simulink model "ScenarioAnalysis"  (R2022a)
settings: Solver=FixedStepDiscrete  StartTime=0.0  StopTime=10.0  RelTol=1e-3
model workspace (MAT data in the model file):
  firstWarning = 1
  originalScenarioChecksum = '40B3C482BC2D2C68EC305C2064A27088'
libraries: drivingscenarioandsensors x2
settings Model: Creator=Jim T  LastModifiedBy=11064

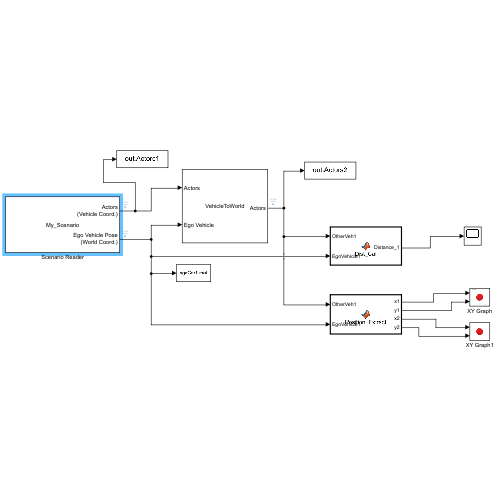
[thumbnail: Simulink's stored preview of the top-level diagram]
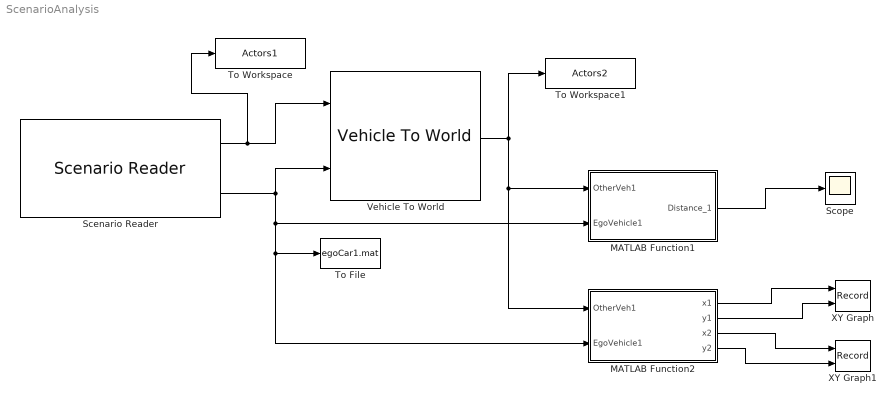
== system ScenarioAnalysis ==
  MATLAB Function1 : MATLAB Function  TreatAsAtomicUnit=on
  MATLAB Function2 : MATLAB Function  TreatAsAtomicUnit=on
  Scenario Reader : drivingscenarioandsensors/Scenario Reader  ScenarioSource=From file  ScenarioFileName=My_Scenario.mat  ScenarioVariableName=scenario  OutputCoordinateSystem=Vehicle coordinates  EgoVehicleSource=Scenario  EgoVehicleActorID=1  OrientVehiclesOnRoad=off  OutputEgoVehiclePose=on  OutputEgoVehicleState=off  SampleTime=0.1  LaneBoundaryOutput=None  LaneBoundaryDistance=0:0.5:9.5  LaneBoundaryLocation=Center of lane markings  BusNameSource=Auto  BusName=BusActors  BusNumActorsSource=Scenario  BusNumActors=100  BusName2Source=Auto  BusName2=BusLaneBoundaries  BusNumLaneBoundariesSource=Scenario  BusNumLaneBoundaries=10  BusName3Source=Auto  BusName3=BusEgoActor  BusName4Source=Auto  BusName4=BusEgoState  ShowCoordinateLabels=on  SimulateUsing=Interpreted execution
  Scope : Scope
  To File : ToFile  Filename=egoCar1.mat  SaveFormat=Timeseries
  To Workspace : ToWorkspace  VariableName=Actors1  SaveFormat=Timeseries  SampleTime=-1
  To Workspace1 : ToWorkspace  VariableName=Actors2  SaveFormat=Timeseries  SampleTime=-1
  Vehicle To World : drivingscenarioandsensors/Vehicle To World  BusNameSource=Auto  BusName=BusVehicleToWorldActors  SimulateUsing=Interpreted execution
      settings: SourceProductBaseCode=DR
  XY Graph : Record  FileSettingsInternal="{\"entries\":[{\"content\":{\"excelSettings\":{\"content\":{},\"type\":\"Streamout.ExcelSettings\"}},\"type\":\"Streamout.FileSettingStorage\",\"uuid\":\"b51cf517-17e0-4542-acce-b7d9d2cd1a5a\"}],\"packageUris\":[\"http://schema.mathworks.com/mf0/streamout_blocks/R2020a\"],\"version\":\"1.0\"}"  Layout=[1 1]  SignalsInternal="{\"entries\":[{\"content\":{\"signals\":[{\"content\":{\"blockPath\":[\"ScenarioAnalysis/XY Graph\"],\"channel\":[],\"dimensions\":[1],\"domain\":\"ScenarioAnalysis/XY Graph\",\"lineColor\":\"#a2142f\",\"plots\":[1],\"port\":1,\"sid\":[],\"signalID\":35,\"signalName\":\"MATLAB Function2:1\"},\"type\":\"RecordBlkView.Signal\",\"uuid\":\"04b8474e-6d3d-4901-9223-983ad539c10e\"},{\"content\":{\"blockPath\":[\"ScenarioAnalysis/XY Graph\"],\"channel\":[],\"dimensions\":[1],\"domain\":\"ScenarioAnalysis/XY Graph\",\"lineColor\":\"#139fff\",\"plots\":[1],\"port\":2,\"sid\":[],\"signalID\":38,\"signalName\":\"MATLAB Function2:2\"},\"type\":\"RecordBlkView.Signal\",\"uuid\":\"012edd8f-518d-447d-b22c-72d910c1f49f\"}]},\"type\":\"RecordBlkView.InputSignals\",\"uuid\":\"3fa3c5aa-3a4d-44aa-9af0-7d29b792f97e\"}],\"packageUris\":[\"http://schema.mathworks.com/mf0/streamout_blocks/R2020a\"],\"version\":\"1.0\"}"  VisualizationBindings="{\"xyplotplugin\":{\"info\":[{\"series\":[{\"bindingParametersList\":[{\"parameter\":\"X-Axis\",\"signalID\":35,\"signalName\":\"MATLAB Function2:1\"},{\"parameter\":\"Y-Axis\",\"signalID\":38,\"signalName\":\"MATLAB Function2:2\"}],\"seriesID\":38687}],\"subplotID\":1}]}}"  CompatibilityTag=XY
  XY Graph1 : Record  FileSettingsInternal="{\"entries\":[{\"content\":{\"excelSettings\":{\"content\":{},\"type\":\"Streamout.ExcelSettings\"}},\"type\":\"Streamout.FileSettingStorage\",\"uuid\":\"6fa187cc-d8dd-4e57-b1e9-641f2adc0ef9\"}],\"packageUris\":[\"http://schema.mathworks.com/mf0/streamout_blocks/R2020a\"],\"version\":\"1.0\"}"  Layout=[1 1]  SignalsInternal="{\"entries\":[{\"content\":{\"signals\":[{\"content\":{\"blockPath\":[\"ScenarioAnalysis/XY Graph1\"],\"channel\":[],\"dimensions\":[1],\"domain\":\"ScenarioAnalysis/XY Graph1\",\"lineColor\":\"#a2142f\",\"plots\":[1],\"port\":1,\"sid\":[],\"signalID\":27,\"signalName\":\"MATLAB Function2:3\"},\"type\":\"RecordBlkView.Signal\",\"uuid\":\"58223eaa-ceba-43fe-afc1-79236a0d2be0\"},{\"content\":{\"blockPath\":[\"ScenarioAnalysis/XY Graph1\"],\"channel\":[],\"dimensions\":[1],\"domain\":\"ScenarioAnalysis/XY Graph1\",\"lineColor\":\"#139fff\",\"plots\":[1],\"port\":2,\"sid\":[],\"signalID\":30,\"signalName\":\"MATLAB Function2:4\"},\"type\":\"RecordBlkView.Signal\",\"uuid\":\"fbcb8779-51c4-4b8c-a218-ba71a7bb535f\"}]},\"type\":\"RecordBlkView.InputSignals\",\"uuid\":\"ed91af77-e76b-4a3b-bc1d-f4c2900ec38e\"}],\"packageUris\":[\"http://schema.mathworks.com/mf0/streamout_blocks/R2020a\"],\"version\":\"1.0\"}"  VisualizationBindings="{\"xyplotplugin\":{\"info\":[{\"series\":[{\"bindingParametersList\":[{\"parameter\":\"X-Axis\",\"signalID\":27,\"signalName\":\"MATLAB Function2:3\"},{\"parameter\":\"Y-Axis\",\"signalID\":30,\"signalName\":\"MATLAB Function2:4\"}],\"seriesID\":22770}],\"subplotID\":1}]}}"  CompatibilityTag=XY
  wires:
  Scenario Reader/1 -> To Workspace/1, Vehicle To World/1
  MATLAB Function1/1(Distance_1) -> Scope/1
  MATLAB Function2/1(x1) -> XY Graph/1
  Vehicle To World/1 -> MATLAB Function2/1(OtherVeh1), MATLAB Function1/1(OtherVeh1), To Workspace1/1
  Scenario Reader/2 -> MATLAB Function1/2(EgoVehicle1), MATLAB Function2/2(EgoVehicle1), To File/1, Vehicle To World/2
  MATLAB Function2/2(y1) -> XY Graph/2
  MATLAB Function2/3(x2) -> XY Graph1/1
  MATLAB Function2/4(y2) -> XY Graph1/2

== matlab function ScenarioAnalysis/MATLAB Function2 ==
  data: OtherVeh1 input; EgoVehicle1 input; x1 output; y1 output; x2 output; y2 output
function [x1,y1,x2,y2] = Position_Extract (OtherVeh1, EgoVehicle1)


x1=OtherVeh1.Actors.Position(:,1);
y1=OtherVeh1.Actors.Position(:,2);

x2=EgoVehicle1.Position(:,1);
y2=EgoVehicle1.Position(:,2);

== matlab function ScenarioAnalysis/MATLAB Function1 ==
  data: OtherVeh1 input; EgoVehicle1 input; Distance_1 output
function Distance_1 = Dist_Cal (OtherVeh1, EgoVehicle1)


x1=OtherVeh1.Actors.Position(:,1);
y1=OtherVeh1.Actors.Position(:,2);

x2=EgoVehicle1.Position(:,1);
y2=EgoVehicle1.Position(:,2);



Distance_1=sqrt((x1-x2)^2+(y1-y2)^2);
